simulink model "CSE_Lab3_No1_Simulink"  (R2023b)
settings: Solver=VariableStepAuto  StartTime=0.0  StopTime=20  RelTol=1e-3
values from neighbouring files (symbols this model uses):
  G1_den = [1 0 0]    [CSE_Lab3_No1_Diagram.m]    (also in CSE_Lab3_No1_ReducedBlockDiagram.m; CSE_Lab3_No2_Matlab.m)
  G1_num = [1]    [CSE_Lab3_No1_Diagram.m]    (also in CSE_Lab3_No1_ReducedBlockDiagram.m; CSE_Lab3_No2_Matlab.m = 1)
  G2_den = [1 1]    [CSE_Lab3_No1_Diagram.m]    (also in CSE_Lab3_No1_ReducedBlockDiagram.m; CSE_Lab3_No2_Matlab.m)
  G2_num = [1]    [CSE_Lab3_No1_Diagram.m]    (also in CSE_Lab3_No1_ReducedBlockDiagram.m; CSE_Lab3_No2_Matlab.m = 1)
  G3_den = [1 0]    [CSE_Lab3_No1_Diagram.m]    (also in CSE_Lab3_No1_ReducedBlockDiagram.m; CSE_Lab3_No2_Matlab.m)
  G3_num = [1]    [CSE_Lab3_No1_Diagram.m]    (also in CSE_Lab3_No1_ReducedBlockDiagram.m; CSE_Lab3_No2_Matlab.m = 1)
  G4_den = [2 0]    [CSE_Lab3_No2_Matlab.m]
  G4_num = 1    [CSE_Lab3_No2_Matlab.m]
  H1_den = [1 0]    [CSE_Lab3_No1_Diagram.m]    (also in CSE_Lab3_No1_ReducedBlockDiagram.m; CSE_Lab3_No2_Matlab.m)
  H1_num = [1]    [CSE_Lab3_No1_Diagram.m]    (also in CSE_Lab3_No1_ReducedBlockDiagram.m; CSE_Lab3_No2_Matlab.m = 1)
  H2_den = [1 -1]    [CSE_Lab3_No1_Diagram.m]    (also in CSE_Lab3_No1_ReducedBlockDiagram.m; CSE_Lab3_No2_Matlab.m)
  H2_num = [1]    [CSE_Lab3_No1_Diagram.m]    (also in CSE_Lab3_No1_ReducedBlockDiagram.m; CSE_Lab3_No2_Matlab.m = 1)
  H3_den = [1 -2]    [CSE_Lab3_No1_Diagram.m]    (also in CSE_Lab3_No1_ReducedBlockDiagram.m; CSE_Lab3_No2_Matlab.m)
  H3_num = [1]    [CSE_Lab3_No1_Diagram.m]    (also in CSE_Lab3_No1_ReducedBlockDiagram.m; CSE_Lab3_No2_Matlab.m = 1)
  TF_6_den = conv(G1G2G3G4_den,TF_6_den_sum)    [CSE_Lab3_No2_Matlab.m]
  TF_6_num = conv(TF_5_num,G1G2G3G4H1_den)    [CSE_Lab3_No2_Matlab.m]
settings Model: Creator=Zolo  LastModifiedBy=Zolo

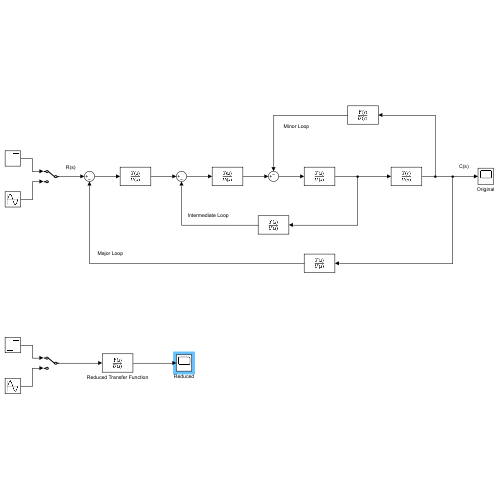
[thumbnail: Simulink's stored preview of the top-level diagram]
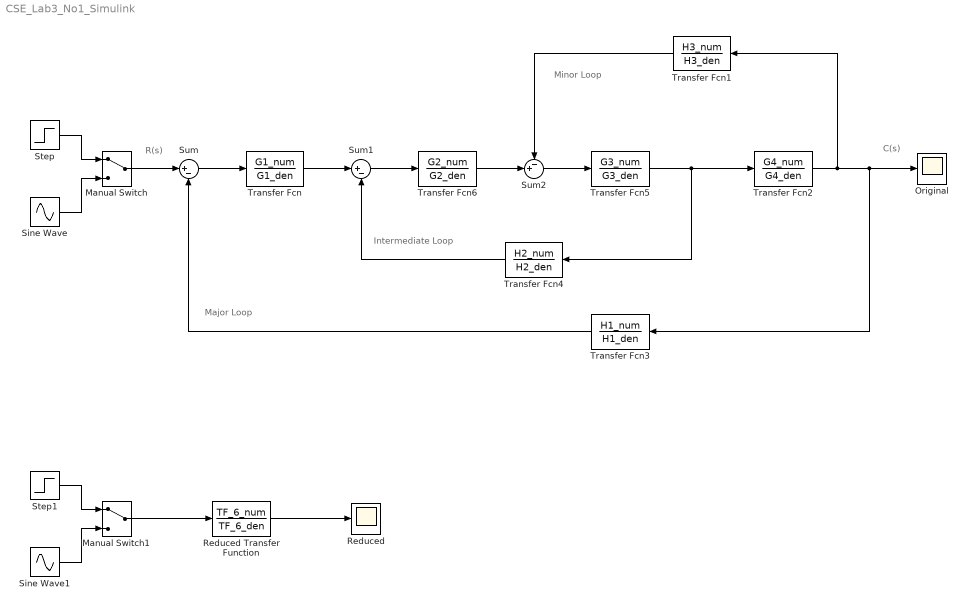
== system CSE_Lab3_No1_Simulink ==
  note: C(s)
  note: R(s)
  note: Major Loop
  note: Intermediate Loop
  note: Minor Loop
  Manual Switch : ManualSwitch
  Manual Switch1 : ManualSwitch
  Original : Scope
  Reduced : Scope
  Reduced Transfer Function : TransferFcn  Numerator=TF_6_num  Denominator=TF_6_den
  Sine Wave : Sin  SampleTime=0
  Sine Wave1 : Sin  SampleTime=0
  Step : Step  SampleTime=0
  Step1 : Step  SampleTime=0
  Sum : Sum  Inputs=|+-
  Sum1 : Sum  Inputs=|+-
  Sum2 : Sum  Inputs=-+|
  Transfer Fcn : TransferFcn  Numerator=G1_num  Denominator=G1_den
  Transfer Fcn1 : TransferFcn  Numerator=H3_num  Denominator=H3_den
  Transfer Fcn2 : TransferFcn  Numerator=G4_num  Denominator=G4_den
  Transfer Fcn3 : TransferFcn  Numerator=H1_num  Denominator=H1_den
  Transfer Fcn4 : TransferFcn  Numerator=H2_num  Denominator=H2_den
  Transfer Fcn5 : TransferFcn  Numerator=G3_num  Denominator=G3_den
  Transfer Fcn6 : TransferFcn  Numerator=G2_num  Denominator=G2_den
  wires:
  Step/1 -> Manual Switch/1
  Sine Wave/1 -> Manual Switch/2
  Manual Switch/1 -> Sum/1
  Sum/1 -> Transfer Fcn/1
  Transfer Fcn/1 -> Sum1/1
  Sum1/1 -> Transfer Fcn6/1
  Sum2/1 -> Transfer Fcn5/1
  Transfer Fcn5/1 -> Transfer Fcn4/1, Transfer Fcn2/1
  Transfer Fcn2/1 -> Transfer Fcn1/1, Transfer Fcn3/1, Original/1
  Transfer Fcn1/1 -> Sum2/1
  Transfer Fcn6/1 -> Sum2/2
  Transfer Fcn4/1 -> Sum1/2
  Transfer Fcn3/1 -> Sum/2
  Sine Wave1/1 -> Manual Switch1/2
  Step1/1 -> Manual Switch1/1
  Manual Switch1/1 -> Reduced Transfer Function/1
  Reduced Transfer Function/1 -> Reduced/1
